simulink model "System3"  (R2025a)
settings: Solver=ode113  StartTime=0.0  StopTime=400  FixedStep=0.01  MaxStep=0.1  RelTol=1e-3
libraries: simulink x3784, slpidlib x2
(part 4 of 160)

== system System3/Battery1/Module3/SubModule_6 ==
  Module_Current : Inport
  Add : Sum  Inputs=++++++++++++++++++++++
  Add1 : Sum  Inputs=++++++++++++++++++++++
  Cell1 : Subsystem
  Cell10 : Subsystem
  Cell11 : Subsystem
  Cell12 : Subsystem
  Cell13 : Subsystem
  Cell14 : Subsystem
  Cell15 : Subsystem
  Cell16 : Subsystem
  Cell17 : Subsystem
  Cell18 : Subsystem
  Cell19 : Subsystem
  Cell2 : Subsystem
  Cell20 : Subsystem
  Cell21 : Subsystem
  Cell22 : Subsystem
  Cell3 : Subsystem
  Cell4 : Subsystem
  Cell5 : Subsystem
  Cell6 : Subsystem
  Cell7 : Subsystem
  Cell8 : Subsystem
  Cell9 : Subsystem
  Constant : Constant  Value=22
  Divide : Product  Inputs=*/
  SubModule_Voltage : Outport
  SubModule_avg_temp : Outport  Port=2
  wires:
  Cell9/2(Cell_temp) -> Add1/9
  [Cell_Current] -> Cell8/1(Cell_Current)
  Cell13/1(Cell_Voltage) -> Add/13
  Cell4/1(Cell_Voltage) -> Add/4
  Module_Current/1 -> [Cell_Current]
  Cell15/1(Cell_Voltage) -> Add/15
  [Cell_Current] -> Cell7/1(Cell_Current)
  [Cell_Current] -> Cell10/1(Cell_Current)
  Cell21/2(Cell_temp) -> Add1/21
  Cell5/1(Cell_Voltage) -> Add/5
  [Cell_Current] -> Cell1/1(Cell_Current)
  Cell2/1(Cell_Voltage) -> Add/2
  Cell19/1(Cell_Voltage) -> Add/19
  [Cell_Current] -> Cell5/1(Cell_Current)
  [Cell_Current] -> Cell11/1(Cell_Current)
  Cell6/1(Cell_Voltage) -> Add/6
  Cell11/1(Cell_Voltage) -> Add/11
  [Cell_Current] -> Cell18/1(Cell_Current)
  Cell7/2(Cell_temp) -> Add1/7
  [Cell_Current] -> Cell21/1(Cell_Current)
  [Cell_Current] -> Cell12/1(Cell_Current)
  [Cell_Current] -> Cell4/1(Cell_Current)
  Cell18/1(Cell_Voltage) -> Add/18
  Cell20/1(Cell_Voltage) -> Add/20
  Cell11/2(Cell_temp) -> Add1/11
  [Cell_Current] -> Cell2/1(Cell_Current)
  Cell16/2(Cell_temp) -> Add1/16
  [Cell_Current] -> Cell15/1(Cell_Current)
  [Cell_Current] -> Cell6/1(Cell_Current)
  [Cell_Current] -> Cell13/1(Cell_Current)
  Cell2/2(Cell_temp) -> Add1/2
  Cell22/2(Cell_temp) -> Add1/22
  Cell9/1(Cell_Voltage) -> Add/9
  Cell7/1(Cell_Voltage) -> Add/7
  [Cell_Current] -> Cell9/1(Cell_Current)
  Cell14/2(Cell_temp) -> Add1/14
  Cell17/1(Cell_Voltage) -> Add/17
  Cell10/2(Cell_temp) -> Add1/10
  [Cell_Current] -> Cell16/1(Cell_Current)
  Cell8/1(Cell_Voltage) -> Add/8
  Cell21/1(Cell_Voltage) -> Add/21
  Cell12/2(Cell_temp) -> Add1/12
  Cell22/1(Cell_Voltage) -> Add/22
  [Cell_Current] -> Cell20/1(Cell_Current)
  [Cell_Current] -> Cell17/1(Cell_Current)
  Cell10/1(Cell_Voltage) -> Add/10
  Cell18/2(Cell_temp) -> Add1/18
  Cell14/1(Cell_Voltage) -> Add/14
  Cell16/1(Cell_Voltage) -> Add/16
  [Cell_Current] -> Cell3/1(Cell_Current)
  Cell12/1(Cell_Voltage) -> Add/12
  Cell20/2(Cell_temp) -> Add1/20
  Cell1/1(Cell_Voltage) -> Add/1
  [Cell_Current] -> Cell19/1(Cell_Current)
  Cell3/1(Cell_Voltage) -> Add/3
  [Cell_Current] -> Cell22/1(Cell_Current)
  [Cell_Current] -> Cell14/1(Cell_Current)
  Cell19/2(Cell_temp) -> Add1/19
  Cell6/2(Cell_temp) -> Add1/6
  Cell17/2(Cell_temp) -> Add1/17
  Cell15/2(Cell_temp) -> Add1/15
  Cell8/2(Cell_temp) -> Add1/8
  Cell3/2(Cell_temp) -> Add1/3
  Cell13/2(Cell_temp) -> Add1/13
  Add/1 -> SubModule_Voltage/1
  Cell4/2(Cell_temp) -> Add1/4
  Cell5/2(Cell_temp) -> Add1/5
  Cell1/2(Cell_temp) -> Add1/1
  Add1/1 -> Divide/1
  Constant/1 -> Divide/2
  Divide/1 -> SubModule_avg_temp/1

== system System3/Battery1/Module3/SubModule_7 ==
  Module_Current : Inport
  Add : Sum  Inputs=++++++++++++++++++++++
  Add1 : Sum  Inputs=++++++++++++++++++++++
  Cell1 : Subsystem
  Cell10 : Subsystem
  Cell11 : Subsystem
  Cell12 : Subsystem
  Cell13 : Subsystem
  Cell14 : Subsystem
  Cell15 : Subsystem
  Cell16 : Subsystem
  Cell17 : Subsystem
  Cell18 : Subsystem
  Cell19 : Subsystem
  Cell2 : Subsystem
  Cell20 : Subsystem
  Cell21 : Subsystem
  Cell22 : Subsystem
  Cell3 : Subsystem
  Cell4 : Subsystem
  Cell5 : Subsystem
  Cell6 : Subsystem
  Cell7 : Subsystem
  Cell8 : Subsystem
  Cell9 : Subsystem
  Constant : Constant  Value=22
  Divide : Product  Inputs=*/
  SubModule_Voltage : Outport
  SubModule_avg_temp : Outport  Port=2
  wires:
  Cell9/2(Cell_temp) -> Add1/9
  [Cell_Current] -> Cell8/1(Cell_Current)
  Cell13/1(Cell_Voltage) -> Add/13
  Cell4/1(Cell_Voltage) -> Add/4
  Module_Current/1 -> [Cell_Current]
  Cell15/1(Cell_Voltage) -> Add/15
  [Cell_Current] -> Cell7/1(Cell_Current)
  [Cell_Current] -> Cell10/1(Cell_Current)
  Cell21/2(Cell_temp) -> Add1/21
  Cell5/1(Cell_Voltage) -> Add/5
  [Cell_Current] -> Cell1/1(Cell_Current)
  Cell2/1(Cell_Voltage) -> Add/2
  Cell19/1(Cell_Voltage) -> Add/19
  [Cell_Current] -> Cell5/1(Cell_Current)
  [Cell_Current] -> Cell11/1(Cell_Current)
  Cell6/1(Cell_Voltage) -> Add/6
  Cell11/1(Cell_Voltage) -> Add/11
  [Cell_Current] -> Cell18/1(Cell_Current)
  Cell7/2(Cell_temp) -> Add1/7
  [Cell_Current] -> Cell21/1(Cell_Current)
  [Cell_Current] -> Cell12/1(Cell_Current)
  [Cell_Current] -> Cell4/1(Cell_Current)
  Cell18/1(Cell_Voltage) -> Add/18
  Cell20/1(Cell_Voltage) -> Add/20
  Cell11/2(Cell_temp) -> Add1/11
  [Cell_Current] -> Cell2/1(Cell_Current)
  Cell16/2(Cell_temp) -> Add1/16
  [Cell_Current] -> Cell15/1(Cell_Current)
  [Cell_Current] -> Cell6/1(Cell_Current)
  [Cell_Current] -> Cell13/1(Cell_Current)
  Cell2/2(Cell_temp) -> Add1/2
  Cell22/2(Cell_temp) -> Add1/22
  Cell9/1(Cell_Voltage) -> Add/9
  Cell7/1(Cell_Voltage) -> Add/7
  [Cell_Current] -> Cell9/1(Cell_Current)
  Cell14/2(Cell_temp) -> Add1/14
  Cell17/1(Cell_Voltage) -> Add/17
  Cell10/2(Cell_temp) -> Add1/10
  [Cell_Current] -> Cell16/1(Cell_Current)
  Cell8/1(Cell_Voltage) -> Add/8
  Cell21/1(Cell_Voltage) -> Add/21
  Cell12/2(Cell_temp) -> Add1/12
  Cell22/1(Cell_Voltage) -> Add/22
  [Cell_Current] -> Cell20/1(Cell_Current)
  [Cell_Current] -> Cell17/1(Cell_Current)
  Cell10/1(Cell_Voltage) -> Add/10
  Cell18/2(Cell_temp) -> Add1/18
  Cell14/1(Cell_Voltage) -> Add/14
  Cell16/1(Cell_Voltage) -> Add/16
  [Cell_Current] -> Cell3/1(Cell_Current)
  Cell12/1(Cell_Voltage) -> Add/12
  Cell20/2(Cell_temp) -> Add1/20
  Cell1/1(Cell_Voltage) -> Add/1
  [Cell_Current] -> Cell19/1(Cell_Current)
  Cell3/1(Cell_Voltage) -> Add/3
  [Cell_Current] -> Cell22/1(Cell_Current)
  [Cell_Current] -> Cell14/1(Cell_Current)
  Cell19/2(Cell_temp) -> Add1/19
  Cell6/2(Cell_temp) -> Add1/6
  Cell17/2(Cell_temp) -> Add1/17
  Cell15/2(Cell_temp) -> Add1/15
  Cell8/2(Cell_temp) -> Add1/8
  Cell3/2(Cell_temp) -> Add1/3
  Cell13/2(Cell_temp) -> Add1/13
  Add/1 -> SubModule_Voltage/1
  Cell4/2(Cell_temp) -> Add1/4
  Cell5/2(Cell_temp) -> Add1/5
  Cell1/2(Cell_temp) -> Add1/1
  Add1/1 -> Divide/1
  Constant/1 -> Divide/2
  Divide/1 -> SubModule_avg_temp/1

== system System3/Battery1/Module3/SubModule_8 ==
  Module_Current : Inport
  Add : Sum  Inputs=++++++++++++++++++++++
  Add1 : Sum  Inputs=++++++++++++++++++++++
  Cell1 : Subsystem
  Cell10 : Subsystem
  Cell11 : Subsystem
  Cell12 : Subsystem
  Cell13 : Subsystem
  Cell14 : Subsystem
  Cell15 : Subsystem
  Cell16 : Subsystem
  Cell17 : Subsystem
  Cell18 : Subsystem
  Cell19 : Subsystem
  Cell2 : Subsystem
  Cell20 : Subsystem
  Cell21 : Subsystem
  Cell22 : Subsystem
  Cell3 : Subsystem
  Cell4 : Subsystem
  Cell5 : Subsystem
  Cell6 : Subsystem
  Cell7 : Subsystem
  Cell8 : Subsystem
  Cell9 : Subsystem
  Constant : Constant  Value=22
  Divide : Product  Inputs=*/
  SubModule_Voltage : Outport
  SubModule_avg_temp : Outport  Port=2
  wires:
  Divide/1 -> SubModule_avg_temp/1
  Constant/1 -> Divide/2
  Add1/1 -> Divide/1
  Cell1/2(Cell_temp) -> Add1/1
  Cell5/2(Cell_temp) -> Add1/5
  Cell4/2(Cell_temp) -> Add1/4
  Add/1 -> SubModule_Voltage/1
  Cell13/2(Cell_temp) -> Add1/13
  Cell3/2(Cell_temp) -> Add1/3
  Cell8/2(Cell_temp) -> Add1/8
  Cell15/2(Cell_temp) -> Add1/15
  Cell17/2(Cell_temp) -> Add1/17
  Cell6/2(Cell_temp) -> Add1/6
  Cell19/2(Cell_temp) -> Add1/19
  [Cell_Current] -> Cell14/1(Cell_Current)
  [Cell_Current] -> Cell22/1(Cell_Current)
  Cell3/1(Cell_Voltage) -> Add/3
  [Cell_Current] -> Cell19/1(Cell_Current)
  Cell1/1(Cell_Voltage) -> Add/1
  Cell20/2(Cell_temp) -> Add1/20
  Cell12/1(Cell_Voltage) -> Add/12
  [Cell_Current] -> Cell3/1(Cell_Current)
  Cell16/1(Cell_Voltage) -> Add/16
  Cell14/1(Cell_Voltage) -> Add/14
  Cell18/2(Cell_temp) -> Add1/18
  Cell10/1(Cell_Voltage) -> Add/10
  [Cell_Current] -> Cell17/1(Cell_Current)
  [Cell_Current] -> Cell20/1(Cell_Current)
  Cell22/1(Cell_Voltage) -> Add/22
  Cell12/2(Cell_temp) -> Add1/12
  Cell21/1(Cell_Voltage) -> Add/21
  Cell8/1(Cell_Voltage) -> Add/8
  [Cell_Current] -> Cell16/1(Cell_Current)
  Cell10/2(Cell_temp) -> Add1/10
  Cell17/1(Cell_Voltage) -> Add/17
  Cell14/2(Cell_temp) -> Add1/14
  [Cell_Current] -> Cell9/1(Cell_Current)
  Cell7/1(Cell_Voltage) -> Add/7
  Cell9/1(Cell_Voltage) -> Add/9
  Cell22/2(Cell_temp) -> Add1/22
  Cell2/2(Cell_temp) -> Add1/2
  [Cell_Current] -> Cell13/1(Cell_Current)
  [Cell_Current] -> Cell6/1(Cell_Current)
  [Cell_Current] -> Cell15/1(Cell_Current)
  Cell16/2(Cell_temp) -> Add1/16
  [Cell_Current] -> Cell2/1(Cell_Current)
  Cell11/2(Cell_temp) -> Add1/11
  Cell20/1(Cell_Voltage) -> Add/20
  Cell18/1(Cell_Voltage) -> Add/18
  [Cell_Current] -> Cell4/1(Cell_Current)
  [Cell_Current] -> Cell12/1(Cell_Current)
  [Cell_Current] -> Cell21/1(Cell_Current)
  Cell7/2(Cell_temp) -> Add1/7
  [Cell_Current] -> Cell18/1(Cell_Current)
  Cell11/1(Cell_Voltage) -> Add/11
  Cell6/1(Cell_Voltage) -> Add/6
  [Cell_Current] -> Cell11/1(Cell_Current)
  [Cell_Current] -> Cell5/1(Cell_Current)
  Cell19/1(Cell_Voltage) -> Add/19
  Cell2/1(Cell_Voltage) -> Add/2
  [Cell_Current] -> Cell1/1(Cell_Current)
  Cell5/1(Cell_Voltage) -> Add/5
  Cell21/2(Cell_temp) -> Add1/21
  [Cell_Current] -> Cell10/1(Cell_Current)
  [Cell_Current] -> Cell7/1(Cell_Current)
  Cell15/1(Cell_Voltage) -> Add/15
  Module_Current/1 -> [Cell_Current]
  Cell4/1(Cell_Voltage) -> Add/4
  Cell13/1(Cell_Voltage) -> Add/13
  [Cell_Current] -> Cell8/1(Cell_Current)
  Cell9/2(Cell_temp) -> Add1/9

== system System3/Battery1/Module3/SubModule_9 ==
  Module_Current : Inport
  Add : Sum  Inputs=++++++++++++++++++++++
  Add1 : Sum  Inputs=++++++++++++++++++++++
  Cell1 : Subsystem
  Cell10 : Subsystem
  Cell11 : Subsystem
  Cell12 : Subsystem
  Cell13 : Subsystem
  Cell14 : Subsystem
  Cell15 : Subsystem
  Cell16 : Subsystem
  Cell17 : Subsystem
  Cell18 : Subsystem
  Cell19 : Subsystem
  Cell2 : Subsystem
  Cell20 : Subsystem
  Cell21 : Subsystem
  Cell22 : Subsystem
  Cell3 : Subsystem
  Cell4 : Subsystem
  Cell5 : Subsystem
  Cell6 : Subsystem
  Cell7 : Subsystem
  Cell8 : Subsystem
  Cell9 : Subsystem
  Constant : Constant  Value=22
  Divide : Product  Inputs=*/
  SubModule_Voltage : Outport
  SubModule_avg_temp : Outport  Port=2
  wires:
  Cell9/2(Cell_temp) -> Add1/9
  [Cell_Current] -> Cell8/1(Cell_Current)
  Cell13/1(Cell_Voltage) -> Add/13
  Cell4/1(Cell_Voltage) -> Add/4
  Module_Current/1 -> [Cell_Current]
  Cell15/1(Cell_Voltage) -> Add/15
  [Cell_Current] -> Cell7/1(Cell_Current)
  [Cell_Current] -> Cell10/1(Cell_Current)
  Cell21/2(Cell_temp) -> Add1/21
  Cell5/1(Cell_Voltage) -> Add/5
  [Cell_Current] -> Cell1/1(Cell_Current)
  Cell2/1(Cell_Voltage) -> Add/2
  Cell19/1(Cell_Voltage) -> Add/19
  [Cell_Current] -> Cell5/1(Cell_Current)
  [Cell_Current] -> Cell11/1(Cell_Current)
  Cell6/1(Cell_Voltage) -> Add/6
  Cell11/1(Cell_Voltage) -> Add/11
  [Cell_Current] -> Cell18/1(Cell_Current)
  Cell7/2(Cell_temp) -> Add1/7
  [Cell_Current] -> Cell21/1(Cell_Current)
  [Cell_Current] -> Cell12/1(Cell_Current)
  [Cell_Current] -> Cell4/1(Cell_Current)
  Cell18/1(Cell_Voltage) -> Add/18
  Cell20/1(Cell_Voltage) -> Add/20
  Cell11/2(Cell_temp) -> Add1/11
  [Cell_Current] -> Cell2/1(Cell_Current)
  Cell16/2(Cell_temp) -> Add1/16
  [Cell_Current] -> Cell15/1(Cell_Current)
  [Cell_Current] -> Cell6/1(Cell_Current)
  [Cell_Current] -> Cell13/1(Cell_Current)
  Cell2/2(Cell_temp) -> Add1/2
  Cell22/2(Cell_temp) -> Add1/22
  Cell9/1(Cell_Voltage) -> Add/9
  Cell7/1(Cell_Voltage) -> Add/7
  [Cell_Current] -> Cell9/1(Cell_Current)
  Cell14/2(Cell_temp) -> Add1/14
  Cell17/1(Cell_Voltage) -> Add/17
  Cell10/2(Cell_temp) -> Add1/10
  [Cell_Current] -> Cell16/1(Cell_Current)
  Cell8/1(Cell_Voltage) -> Add/8
  Cell21/1(Cell_Voltage) -> Add/21
  Cell12/2(Cell_temp) -> Add1/12
  Cell22/1(Cell_Voltage) -> Add/22
  [Cell_Current] -> Cell20/1(Cell_Current)
  [Cell_Current] -> Cell17/1(Cell_Current)
  Cell10/1(Cell_Voltage) -> Add/10
  Cell18/2(Cell_temp) -> Add1/18
  Cell14/1(Cell_Voltage) -> Add/14
  Cell16/1(Cell_Voltage) -> Add/16
  [Cell_Current] -> Cell3/1(Cell_Current)
  Cell12/1(Cell_Voltage) -> Add/12
  Cell20/2(Cell_temp) -> Add1/20
  Cell1/1(Cell_Voltage) -> Add/1
  [Cell_Current] -> Cell19/1(Cell_Current)
  Cell3/1(Cell_Voltage) -> Add/3
  [Cell_Current] -> Cell22/1(Cell_Current)
  [Cell_Current] -> Cell14/1(Cell_Current)
  Cell19/2(Cell_temp) -> Add1/19
  Cell6/2(Cell_temp) -> Add1/6
  Cell17/2(Cell_temp) -> Add1/17
  Cell15/2(Cell_temp) -> Add1/15
  Cell8/2(Cell_temp) -> Add1/8
  Cell3/2(Cell_temp) -> Add1/3
  Cell13/2(Cell_temp) -> Add1/13
  Add/1 -> SubModule_Voltage/1
  Cell4/2(Cell_temp) -> Add1/4
  Cell5/2(Cell_temp) -> Add1/5
  Cell1/2(Cell_temp) -> Add1/1
  Add1/1 -> Divide/1
  Constant/1 -> Divide/2
  Divide/1 -> SubModule_avg_temp/1

== system System3/Battery1/SOCEstimator/SOCEstimator ==
  SOC_Initial : Inport
  Current : Inport  Port=2
  CellCapacity : Inport  Port=3
  Add1 : Sum  Inputs=+-
  Constant : Constant  Value=100  SampleTime=-1
  Constant1 : Constant  Value=3600  SampleTime=-1
  Delay : Delay  DelayLength=1  InitialConditionSource=Input port
      settings: InputPortMap=u0,p4
  Divide : Product  Inputs=*//
  Divide1 : Product  Inputs=*/
  Integrator : Integrator
  Saturation1 : Saturate  UpperLimit=1  LowerLimit=0
  SOC : Outport
  wires:
  Add1/1 -> Saturation1/1
  Constant/1 -> Divide1/2
  Divide1/1 -> Delay/2, Add1/1
  Divide/1 -> Add1/2
  Saturation1/1 -> Delay/1
  SOC_Initial/1 -> Divide1/1
  Current/1 -> Integrator/1
  Delay/1 -> SOC/1
  CellCapacity/1 -> Divide/2
  Constant1/1 -> Divide/3
  Integrator/1 -> Divide/1

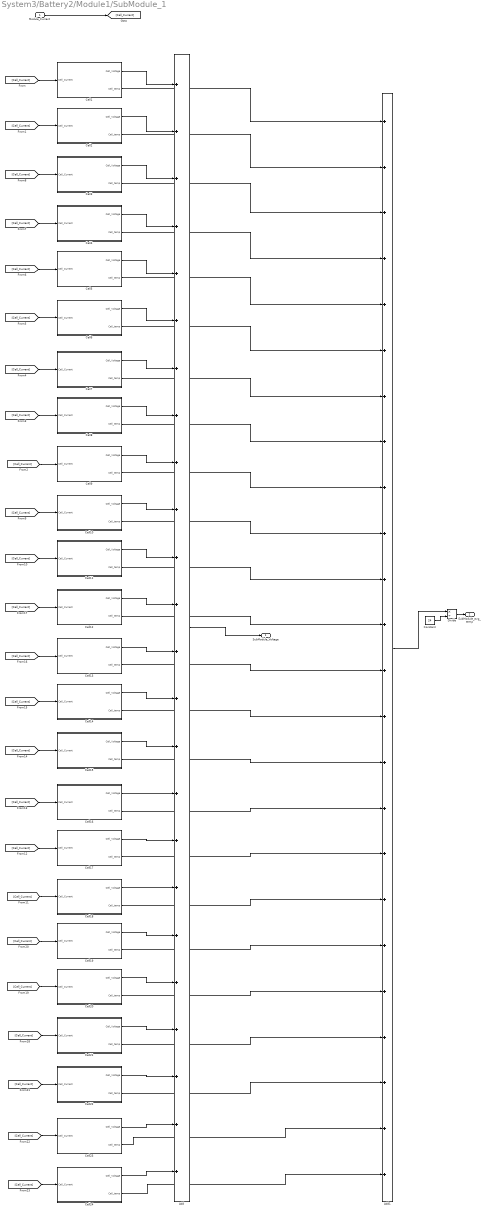
== system System3/Battery2/Module1/SubModule_1 ==
  Module_Current : Inport
  Add : Sum  Inputs=++++++++++++++++++++++++
  Add1 : Sum  Inputs=++++++++++++++++++++++++
  Cell1 : Subsystem
  Cell10 : Subsystem
  Cell11 : Subsystem
  Cell12 : Subsystem
  Cell13 : Subsystem
  Cell14 : Subsystem
  Cell15 : Subsystem
  Cell16 : Subsystem
  Cell17 : Subsystem
  Cell18 : Subsystem
  Cell19 : Subsystem
  Cell2 : Subsystem
  Cell20 : Subsystem
  Cell21 : Subsystem
  Cell22 : Subsystem
  Cell23 : Subsystem
  Cell24 : Subsystem
  Cell3 : Subsystem
  Cell4 : Subsystem
  Cell5 : Subsystem
  Cell6 : Subsystem
  Cell7 : Subsystem
  Cell8 : Subsystem
  Cell9 : Subsystem
  Constant : Constant  Value=24
  Divide : Product  Inputs=*/
  SubModule_Voltage : Outport
  SubModule_avg_temp : Outport  Port=2
  wires:
  Cell9/2(Cell_temp) -> Add1/9
  [Cell_Current] -> Cell8/1(Cell_Current)
  Cell13/1(Cell_Voltage) -> Add/13
  Cell4/1(Cell_Voltage) -> Add/4
  Module_Current/1 -> [Cell_Current]
  Cell15/1(Cell_Voltage) -> Add/15
  [Cell_Current] -> Cell7/1(Cell_Current)
  [Cell_Current] -> Cell10/1(Cell_Current)
  Cell21/2(Cell_temp) -> Add1/21
  Cell5/1(Cell_Voltage) -> Add/5
  [Cell_Current] -> Cell1/1(Cell_Current)
  Cell2/1(Cell_Voltage) -> Add/2
  Cell19/1(Cell_Voltage) -> Add/19
  [Cell_Current] -> Cell5/1(Cell_Current)
  [Cell_Current] -> Cell11/1(Cell_Current)
  Cell6/1(Cell_Voltage) -> Add/6
  Cell11/1(Cell_Voltage) -> Add/11
  [Cell_Current] -> Cell18/1(Cell_Current)
  Cell7/2(Cell_temp) -> Add1/7
  [Cell_Current] -> Cell21/1(Cell_Current)
  [Cell_Current] -> Cell12/1(Cell_Current)
  [Cell_Current] -> Cell4/1(Cell_Current)
  Cell18/1(Cell_Voltage) -> Add/18
  Cell20/1(Cell_Voltage) -> Add/20
  Cell11/2(Cell_temp) -> Add1/11
  [Cell_Current] -> Cell2/1(Cell_Current)
  Cell16/2(Cell_temp) -> Add1/16
  [Cell_Current] -> Cell15/1(Cell_Current)
  [Cell_Current] -> Cell6/1(Cell_Current)
  [Cell_Current] -> Cell13/1(Cell_Current)
  Cell2/2(Cell_temp) -> Add1/2
  Cell22/2(Cell_temp) -> Add1/22
  Cell9/1(Cell_Voltage) -> Add/9
  Cell7/1(Cell_Voltage) -> Add/7
  [Cell_Current] -> Cell9/1(Cell_Current)
  Cell14/2(Cell_temp) -> Add1/14
  Cell17/1(Cell_Voltage) -> Add/17
  Cell10/2(Cell_temp) -> Add1/10
  [Cell_Current] -> Cell16/1(Cell_Current)
  Cell8/1(Cell_Voltage) -> Add/8
  Cell21/1(Cell_Voltage) -> Add/21
  Cell12/2(Cell_temp) -> Add1/12
  Cell22/1(Cell_Voltage) -> Add/22
  [Cell_Current] -> Cell20/1(Cell_Current)
  [Cell_Current] -> Cell17/1(Cell_Current)
  Cell10/1(Cell_Voltage) -> Add/10
  Cell18/2(Cell_temp) -> Add1/18
  Cell14/1(Cell_Voltage) -> Add/14
  Cell16/1(Cell_Voltage) -> Add/16
  [Cell_Current] -> Cell3/1(Cell_Current)
  Cell12/1(Cell_Voltage) -> Add/12
  Cell20/2(Cell_temp) -> Add1/20
  Cell1/1(Cell_Voltage) -> Add/1
  [Cell_Current] -> Cell19/1(Cell_Current)
  Cell3/1(Cell_Voltage) -> Add/3
  [Cell_Current] -> Cell22/1(Cell_Current)
  [Cell_Current] -> Cell14/1(Cell_Current)
  Cell19/2(Cell_temp) -> Add1/19
  Cell6/2(Cell_temp) -> Add1/6
  Cell17/2(Cell_temp) -> Add1/17
  Cell15/2(Cell_temp) -> Add1/15
  Cell8/2(Cell_temp) -> Add1/8
  Cell3/2(Cell_temp) -> Add1/3
  Cell13/2(Cell_temp) -> Add1/13
  Add/1 -> SubModule_Voltage/1
  Cell4/2(Cell_temp) -> Add1/4
  Cell5/2(Cell_temp) -> Add1/5
  Cell1/2(Cell_temp) -> Add1/1
  Add1/1 -> Divide/1
  Constant/1 -> Divide/2
  Divide/1 -> SubModule_avg_temp/1
  [Cell_Current] -> Cell24/1(Cell_Current)
  [Cell_Current] -> Cell23/1(Cell_Current)
  Cell23/1(Cell_Voltage) -> Add/23
  Cell24/1(Cell_Voltage) -> Add/24
  Cell23/2(Cell_temp) -> Add1/23
  Cell24/2(Cell_temp) -> Add1/24

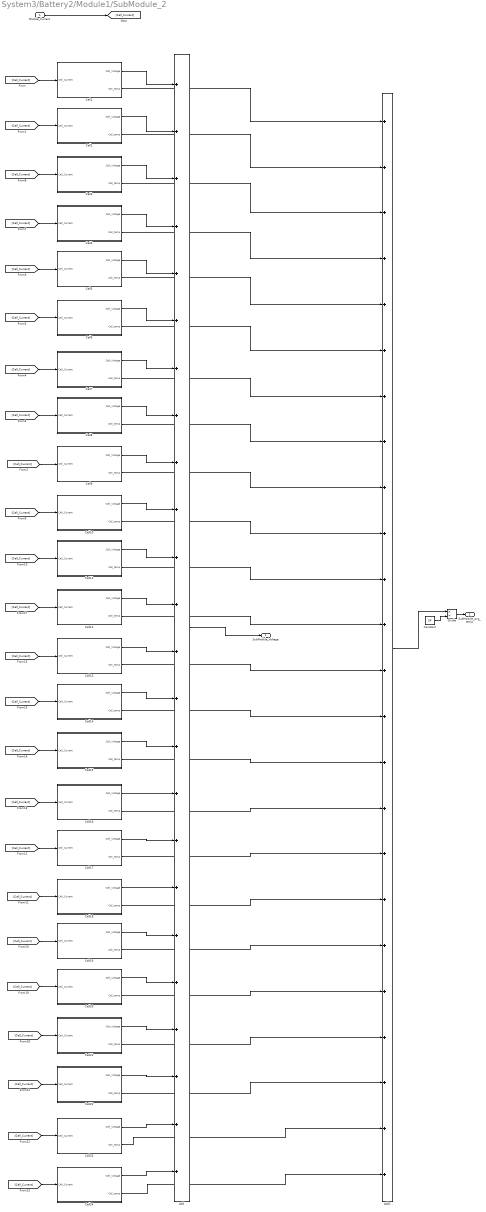
== system System3/Battery2/Module1/SubModule_2 ==
  Module_Current : Inport
  Add : Sum  Inputs=++++++++++++++++++++++++
  Add1 : Sum  Inputs=++++++++++++++++++++++++
  Cell1 : Subsystem
  Cell10 : Subsystem
  Cell11 : Subsystem
  Cell12 : Subsystem
  Cell13 : Subsystem
  Cell14 : Subsystem
  Cell15 : Subsystem
  Cell16 : Subsystem
  Cell17 : Subsystem
  Cell18 : Subsystem
  Cell19 : Subsystem
  Cell2 : Subsystem
  Cell20 : Subsystem
  Cell21 : Subsystem
  Cell22 : Subsystem
  Cell23 : Subsystem
  Cell24 : Subsystem
  Cell3 : Subsystem
  Cell4 : Subsystem
  Cell5 : Subsystem
  Cell6 : Subsystem
  Cell7 : Subsystem
  Cell8 : Subsystem
  Cell9 : Subsystem
  Constant : Constant  Value=24
  Divide : Product  Inputs=*/
  SubModule_Voltage : Outport
  SubModule_avg_temp : Outport  Port=2
  wires:
  Cell24/2(Cell_temp) -> Add1/24
  Cell23/2(Cell_temp) -> Add1/23
  Cell24/1(Cell_Voltage) -> Add/24
  Cell23/1(Cell_Voltage) -> Add/23
  [Cell_Current] -> Cell23/1(Cell_Current)
  [Cell_Current] -> Cell24/1(Cell_Current)
  Divide/1 -> SubModule_avg_temp/1
  Constant/1 -> Divide/2
  Add1/1 -> Divide/1
  Cell1/2(Cell_temp) -> Add1/1
  Cell5/2(Cell_temp) -> Add1/5
  Cell4/2(Cell_temp) -> Add1/4
  Add/1 -> SubModule_Voltage/1
  Cell13/2(Cell_temp) -> Add1/13
  Cell3/2(Cell_temp) -> Add1/3
  Cell8/2(Cell_temp) -> Add1/8
  Cell15/2(Cell_temp) -> Add1/15
  Cell17/2(Cell_temp) -> Add1/17
  Cell6/2(Cell_temp) -> Add1/6
  Cell19/2(Cell_temp) -> Add1/19
  [Cell_Current] -> Cell14/1(Cell_Current)
  [Cell_Current] -> Cell22/1(Cell_Current)
  Cell3/1(Cell_Voltage) -> Add/3
  [Cell_Current] -> Cell19/1(Cell_Current)
  Cell1/1(Cell_Voltage) -> Add/1
  Cell20/2(Cell_temp) -> Add1/20
  Cell12/1(Cell_Voltage) -> Add/12
  [Cell_Current] -> Cell3/1(Cell_Current)
  Cell16/1(Cell_Voltage) -> Add/16
  Cell14/1(Cell_Voltage) -> Add/14
  Cell18/2(Cell_temp) -> Add1/18
  Cell10/1(Cell_Voltage) -> Add/10
  [Cell_Current] -> Cell17/1(Cell_Current)
  [Cell_Current] -> Cell20/1(Cell_Current)
  Cell22/1(Cell_Voltage) -> Add/22
  Cell12/2(Cell_temp) -> Add1/12
  Cell21/1(Cell_Voltage) -> Add/21
  Cell8/1(Cell_Voltage) -> Add/8
  [Cell_Current] -> Cell16/1(Cell_Current)
  Cell10/2(Cell_temp) -> Add1/10
  Cell17/1(Cell_Voltage) -> Add/17
  Cell14/2(Cell_temp) -> Add1/14
  [Cell_Current] -> Cell9/1(Cell_Current)
  Cell7/1(Cell_Voltage) -> Add/7
  Cell9/1(Cell_Voltage) -> Add/9
  Cell22/2(Cell_temp) -> Add1/22
  Cell2/2(Cell_temp) -> Add1/2
  [Cell_Current] -> Cell13/1(Cell_Current)
  [Cell_Current] -> Cell6/1(Cell_Current)
  [Cell_Current] -> Cell15/1(Cell_Current)
  Cell16/2(Cell_temp) -> Add1/16
  [Cell_Current] -> Cell2/1(Cell_Current)
  Cell11/2(Cell_temp) -> Add1/11
  Cell20/1(Cell_Voltage) -> Add/20
  Cell18/1(Cell_Voltage) -> Add/18
  [Cell_Current] -> Cell4/1(Cell_Current)
  [Cell_Current] -> Cell12/1(Cell_Current)
  [Cell_Current] -> Cell21/1(Cell_Current)
  Cell7/2(Cell_temp) -> Add1/7
  [Cell_Current] -> Cell18/1(Cell_Current)
  Cell11/1(Cell_Voltage) -> Add/11
  Cell6/1(Cell_Voltage) -> Add/6
  [Cell_Current] -> Cell11/1(Cell_Current)
  [Cell_Current] -> Cell5/1(Cell_Current)
  Cell19/1(Cell_Voltage) -> Add/19
  Cell2/1(Cell_Voltage) -> Add/2
  [Cell_Current] -> Cell1/1(Cell_Current)
  Cell5/1(Cell_Voltage) -> Add/5
  Cell21/2(Cell_temp) -> Add1/21
  [Cell_Current] -> Cell10/1(Cell_Current)
  [Cell_Current] -> Cell7/1(Cell_Current)
  Cell15/1(Cell_Voltage) -> Add/15
  Module_Current/1 -> [Cell_Current]
  Cell4/1(Cell_Voltage) -> Add/4
  Cell13/1(Cell_Voltage) -> Add/13
  [Cell_Current] -> Cell8/1(Cell_Current)
  Cell9/2(Cell_temp) -> Add1/9

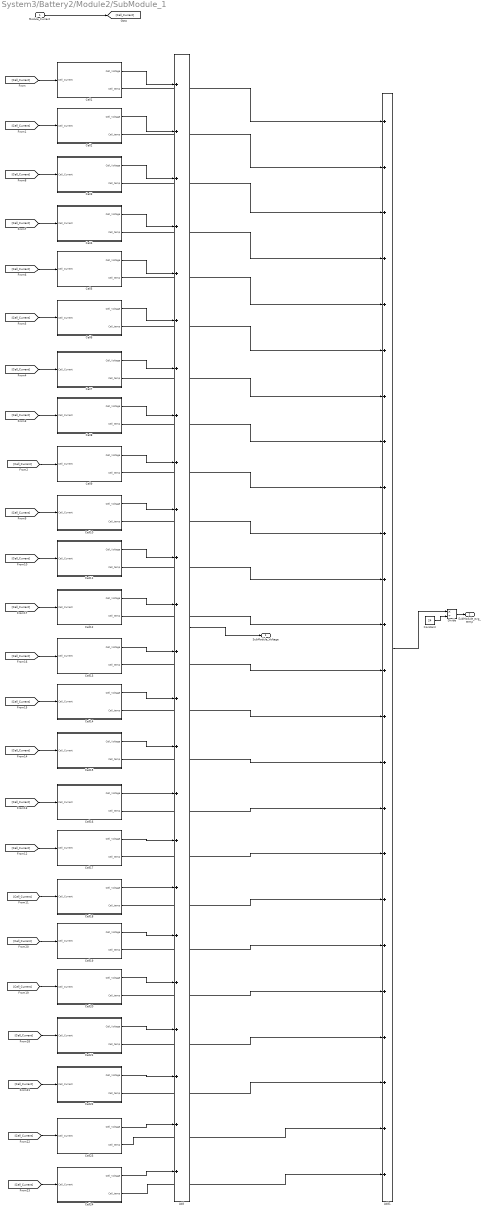
== system System3/Battery2/Module2/SubModule_1 ==
  Module_Current : Inport
  Add : Sum  Inputs=++++++++++++++++++++++++
  Add1 : Sum  Inputs=++++++++++++++++++++++++
  Cell1 : Subsystem
  Cell10 : Subsystem
  Cell11 : Subsystem
  Cell12 : Subsystem
  Cell13 : Subsystem
  Cell14 : Subsystem
  Cell15 : Subsystem
  Cell16 : Subsystem
  Cell17 : Subsystem
  Cell18 : Subsystem
  Cell19 : Subsystem
  Cell2 : Subsystem
  Cell20 : Subsystem
  Cell21 : Subsystem
  Cell22 : Subsystem
  Cell23 : Subsystem
  Cell24 : Subsystem
  Cell3 : Subsystem
  Cell4 : Subsystem
  Cell5 : Subsystem
  Cell6 : Subsystem
  Cell7 : Subsystem
  Cell8 : Subsystem
  Cell9 : Subsystem
  Constant : Constant  Value=24
  Divide : Product  Inputs=*/
  SubModule_Voltage : Outport
  SubModule_avg_temp : Outport  Port=2
  wires:
  Cell24/2(Cell_temp) -> Add1/24
  Cell23/2(Cell_temp) -> Add1/23
  Cell24/1(Cell_Voltage) -> Add/24
  Cell23/1(Cell_Voltage) -> Add/23
  [Cell_Current] -> Cell23/1(Cell_Current)
  [Cell_Current] -> Cell24/1(Cell_Current)
  Divide/1 -> SubModule_avg_temp/1
  Constant/1 -> Divide/2
  Add1/1 -> Divide/1
  Cell1/2(Cell_temp) -> Add1/1
  Cell5/2(Cell_temp) -> Add1/5
  Cell4/2(Cell_temp) -> Add1/4
  Add/1 -> SubModule_Voltage/1
  Cell13/2(Cell_temp) -> Add1/13
  Cell3/2(Cell_temp) -> Add1/3
  Cell8/2(Cell_temp) -> Add1/8
  Cell15/2(Cell_temp) -> Add1/15
  Cell17/2(Cell_temp) -> Add1/17
  Cell6/2(Cell_temp) -> Add1/6
  Cell19/2(Cell_temp) -> Add1/19
  [Cell_Current] -> Cell14/1(Cell_Current)
  [Cell_Current] -> Cell22/1(Cell_Current)
  Cell3/1(Cell_Voltage) -> Add/3
  [Cell_Current] -> Cell19/1(Cell_Current)
  Cell1/1(Cell_Voltage) -> Add/1
  Cell20/2(Cell_temp) -> Add1/20
  Cell12/1(Cell_Voltage) -> Add/12
  [Cell_Current] -> Cell3/1(Cell_Current)
  Cell16/1(Cell_Voltage) -> Add/16
  Cell14/1(Cell_Voltage) -> Add/14
  Cell18/2(Cell_temp) -> Add1/18
  Cell10/1(Cell_Voltage) -> Add/10
  [Cell_Current] -> Cell17/1(Cell_Current)
  [Cell_Current] -> Cell20/1(Cell_Current)
  Cell22/1(Cell_Voltage) -> Add/22
  Cell12/2(Cell_temp) -> Add1/12
  Cell21/1(Cell_Voltage) -> Add/21
  Cell8/1(Cell_Voltage) -> Add/8
  [Cell_Current] -> Cell16/1(Cell_Current)
  Cell10/2(Cell_temp) -> Add1/10
  Cell17/1(Cell_Voltage) -> Add/17
  Cell14/2(Cell_temp) -> Add1/14
  [Cell_Current] -> Cell9/1(Cell_Current)
  Cell7/1(Cell_Voltage) -> Add/7
  Cell9/1(Cell_Voltage) -> Add/9
  Cell22/2(Cell_temp) -> Add1/22
  Cell2/2(Cell_temp) -> Add1/2
  [Cell_Current] -> Cell13/1(Cell_Current)
  [Cell_Current] -> Cell6/1(Cell_Current)
  [Cell_Current] -> Cell15/1(Cell_Current)
  Cell16/2(Cell_temp) -> Add1/16
  [Cell_Current] -> Cell2/1(Cell_Current)
  Cell11/2(Cell_temp) -> Add1/11
  Cell20/1(Cell_Voltage) -> Add/20
  Cell18/1(Cell_Voltage) -> Add/18
  [Cell_Current] -> Cell4/1(Cell_Current)
  [Cell_Current] -> Cell12/1(Cell_Current)
  [Cell_Current] -> Cell21/1(Cell_Current)
  Cell7/2(Cell_temp) -> Add1/7
  [Cell_Current] -> Cell18/1(Cell_Current)
  Cell11/1(Cell_Voltage) -> Add/11
  Cell6/1(Cell_Voltage) -> Add/6
  [Cell_Current] -> Cell11/1(Cell_Current)
  [Cell_Current] -> Cell5/1(Cell_Current)
  Cell19/1(Cell_Voltage) -> Add/19
  Cell2/1(Cell_Voltage) -> Add/2
  [Cell_Current] -> Cell1/1(Cell_Current)
  Cell5/1(Cell_Voltage) -> Add/5
  Cell21/2(Cell_temp) -> Add1/21
  [Cell_Current] -> Cell10/1(Cell_Current)
  [Cell_Current] -> Cell7/1(Cell_Current)
  Cell15/1(Cell_Voltage) -> Add/15
  Module_Current/1 -> [Cell_Current]
  Cell4/1(Cell_Voltage) -> Add/4
  Cell13/1(Cell_Voltage) -> Add/13
  [Cell_Current] -> Cell8/1(Cell_Current)
  Cell9/2(Cell_temp) -> Add1/9

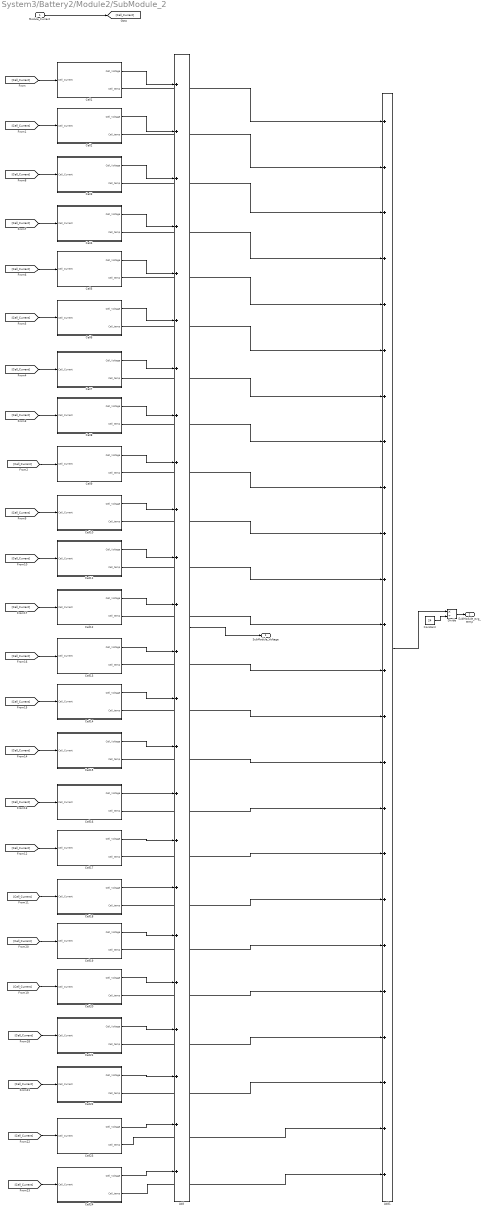
== system System3/Battery2/Module2/SubModule_2 ==
  Module_Current : Inport
  Add : Sum  Inputs=++++++++++++++++++++++++
  Add1 : Sum  Inputs=++++++++++++++++++++++++
  Cell1 : Subsystem
  Cell10 : Subsystem
  Cell11 : Subsystem
  Cell12 : Subsystem
  Cell13 : Subsystem
  Cell14 : Subsystem
  Cell15 : Subsystem
  Cell16 : Subsystem
  Cell17 : Subsystem
  Cell18 : Subsystem
  Cell19 : Subsystem
  Cell2 : Subsystem
  Cell20 : Subsystem
  Cell21 : Subsystem
  Cell22 : Subsystem
  Cell23 : Subsystem
  Cell24 : Subsystem
  Cell3 : Subsystem
  Cell4 : Subsystem
  Cell5 : Subsystem
  Cell6 : Subsystem
  Cell7 : Subsystem
  Cell8 : Subsystem
  Cell9 : Subsystem
  Constant : Constant  Value=24
  Divide : Product  Inputs=*/
  SubModule_Voltage : Outport
  SubModule_avg_temp : Outport  Port=2
  wires:
  Cell9/2(Cell_temp) -> Add1/9
  [Cell_Current] -> Cell8/1(Cell_Current)
  Cell13/1(Cell_Voltage) -> Add/13
  Cell4/1(Cell_Voltage) -> Add/4
  Module_Current/1 -> [Cell_Current]
  Cell15/1(Cell_Voltage) -> Add/15
  [Cell_Current] -> Cell7/1(Cell_Current)
  [Cell_Current] -> Cell10/1(Cell_Current)
  Cell21/2(Cell_temp) -> Add1/21
  Cell5/1(Cell_Voltage) -> Add/5
  [Cell_Current] -> Cell1/1(Cell_Current)
  Cell2/1(Cell_Voltage) -> Add/2
  Cell19/1(Cell_Voltage) -> Add/19
  [Cell_Current] -> Cell5/1(Cell_Current)
  [Cell_Current] -> Cell11/1(Cell_Current)
  Cell6/1(Cell_Voltage) -> Add/6
  Cell11/1(Cell_Voltage) -> Add/11
  [Cell_Current] -> Cell18/1(Cell_Current)
  Cell7/2(Cell_temp) -> Add1/7
  [Cell_Current] -> Cell21/1(Cell_Current)
  [Cell_Current] -> Cell12/1(Cell_Current)
  [Cell_Current] -> Cell4/1(Cell_Current)
  Cell18/1(Cell_Voltage) -> Add/18
  Cell20/1(Cell_Voltage) -> Add/20
  Cell11/2(Cell_temp) -> Add1/11
  [Cell_Current] -> Cell2/1(Cell_Current)
  Cell16/2(Cell_temp) -> Add1/16
  [Cell_Current] -> Cell15/1(Cell_Current)
  [Cell_Current] -> Cell6/1(Cell_Current)
  [Cell_Current] -> Cell13/1(Cell_Current)
  Cell2/2(Cell_temp) -> Add1/2
  Cell22/2(Cell_temp) -> Add1/22
  Cell9/1(Cell_Voltage) -> Add/9
  Cell7/1(Cell_Voltage) -> Add/7
  [Cell_Current] -> Cell9/1(Cell_Current)
  Cell14/2(Cell_temp) -> Add1/14
  Cell17/1(Cell_Voltage) -> Add/17
  Cell10/2(Cell_temp) -> Add1/10
  [Cell_Current] -> Cell16/1(Cell_Current)
  Cell8/1(Cell_Voltage) -> Add/8
  Cell21/1(Cell_Voltage) -> Add/21
  Cell12/2(Cell_temp) -> Add1/12
  Cell22/1(Cell_Voltage) -> Add/22
  [Cell_Current] -> Cell20/1(Cell_Current)
  [Cell_Current] -> Cell17/1(Cell_Current)
  Cell10/1(Cell_Voltage) -> Add/10
  Cell18/2(Cell_temp) -> Add1/18
  Cell14/1(Cell_Voltage) -> Add/14
  Cell16/1(Cell_Voltage) -> Add/16
  [Cell_Current] -> Cell3/1(Cell_Current)
  Cell12/1(Cell_Voltage) -> Add/12
  Cell20/2(Cell_temp) -> Add1/20
  Cell1/1(Cell_Voltage) -> Add/1
  [Cell_Current] -> Cell19/1(Cell_Current)
  Cell3/1(Cell_Voltage) -> Add/3
  [Cell_Current] -> Cell22/1(Cell_Current)
  [Cell_Current] -> Cell14/1(Cell_Current)
  Cell19/2(Cell_temp) -> Add1/19
  Cell6/2(Cell_temp) -> Add1/6
  Cell17/2(Cell_temp) -> Add1/17
  Cell15/2(Cell_temp) -> Add1/15
  Cell8/2(Cell_temp) -> Add1/8
  Cell3/2(Cell_temp) -> Add1/3
  Cell13/2(Cell_temp) -> Add1/13
  Add/1 -> SubModule_Voltage/1
  Cell4/2(Cell_temp) -> Add1/4
  Cell5/2(Cell_temp) -> Add1/5
  Cell1/2(Cell_temp) -> Add1/1
  Add1/1 -> Divide/1
  Constant/1 -> Divide/2
  Divide/1 -> SubModule_avg_temp/1
  [Cell_Current] -> Cell24/1(Cell_Current)
  [Cell_Current] -> Cell23/1(Cell_Current)
  Cell23/1(Cell_Voltage) -> Add/23
  Cell24/1(Cell_Voltage) -> Add/24
  Cell23/2(Cell_temp) -> Add1/23
  Cell24/2(Cell_temp) -> Add1/24

== system System3/Battery2/SOCEstimator/SOCEstimator ==
  SOC_Initial : Inport
  Current : Inport  Port=2
  CellCapacity : Inport  Port=3
  Add1 : Sum  Inputs=+-
  Constant : Constant  Value=100  SampleTime=-1
  Constant1 : Constant  Value=3600  SampleTime=-1
  Delay : Delay  DelayLength=1  InitialConditionSource=Input port
      settings: InputPortMap=u0,p4
  Divide : Product  Inputs=*//
  Divide1 : Product  Inputs=*/
  Integrator : Integrator
  Saturation1 : Saturate  UpperLimit=1  LowerLimit=0
  SOC : Outport
  wires:
  Add1/1 -> Saturation1/1
  Constant/1 -> Divide1/2
  Divide1/1 -> Delay/2, Add1/1
  Divide/1 -> Add1/2
  Saturation1/1 -> Delay/1
  SOC_Initial/1 -> Divide1/1
  Current/1 -> Integrator/1
  Delay/1 -> SOC/1
  CellCapacity/1 -> Divide/2
  Constant1/1 -> Divide/3
  Integrator/1 -> Divide/1

== system System3/Battery1/Module1/SubModule_1/Cell1 ==
  Cell_Current : Inport
  2RC : Subsystem
  Add : Sum  Inputs=---+
  Lookup Table Dynamic2 : simulink/Lookup Tables/Lookup Table Dynamic  LookUpMeth=Interpolation-Use End Values  OutDataType=fixdt('double')  OutScaling=[]  OutputDataTypeScalingMode=Specify via dialog  OutDataTypeStr=fixdt('double')  DoSatur=off
  Product : Product
  Redution_factor : Constant  Value=[0.8 0.85 0.88 0.95 1 0.98 0.95]
  SOCEstimator : Subsystem  TreatAsAtomicUnit=on
  SOC_Mapping : Subsystem
  Scope : Scope
      settings: DataLoggingSaveFormat=Array
  Scope1 : Scope
      settings: DataLoggingVariableName=ScopeData2  DataLoggingSaveFormat=Array
  Scope2 : Scope
      settings: DataLoggingSaveFormat=Array
  Subsystem : Subsystem
  Temp : Constant  Value=[0 10 20 30 40 50 60]
  Cell_Voltage : Outport
  Cell_temp : Outport  Port=2
  wires:
  2RC/2(V2) -> Add/2
  SOC_Mapping/3(C1) -> 2RC/4(C1)
  SOCEstimator/1(SOC) -> SOC_Mapping/1(SOC), Scope/1
  Add/1 -> Scope2/1, Cell_Voltage/1
  SOC_Mapping/1(Ri) -> Subsystem/2(Ri), 2RC/2(Ri)
  2RC/1(V1) -> Add/1
  2RC/3(Vi) -> Add/3
  Cell_Current/1 -> Subsystem/1(Cell_Current), 2RC/1(Current), SOCEstimator/2(Current)
  SOC_Mapping/2(R1) -> 2RC/3(R1)
  [Cell_Capacity] -> Product/1
  SOC_Mapping/5(C2) -> 2RC/6(C2)
  SOC_Mapping/4(R2) -> 2RC/5(R2)
  [SOC_Iinitial] -> SOCEstimator/1(SOC_Initial)
  SOC_Mapping/6(OCV) -> Add/4
  Subsystem/1(Temp_Cell) -> Scope1/1, SOC_Mapping/2(Cell_Temp), Lookup Table Dynamic2/1, Cell_temp/1
  Product/1 -> SOCEstimator/3(Cell_Capacity)
  Lookup Table Dynamic2/1 -> Product/2
  Temp/1 -> Lookup Table Dynamic2/2
  Redution_factor/1 -> Lookup Table Dynamic2/3

== system System3/Battery1/Module1/SubModule_1/Cell10 ==
  Cell_Current : Inport
  2RC : Subsystem
  Add : Sum  Inputs=---+
  Lookup Table Dynamic2 : simulink/Lookup Tables/Lookup Table Dynamic  LookUpMeth=Interpolation-Use End Values  OutDataType=fixdt('double')  OutScaling=[]  OutputDataTypeScalingMode=Specify via dialog  OutDataTypeStr=fixdt('double')  DoSatur=off
  Product : Product
  Redution_factor : Constant  Value=[0.8 0.85 0.88 0.95 1 0.98 0.95]
  SOCEstimator : Subsystem  TreatAsAtomicUnit=on
  SOC_Mapping : Subsystem
  Scope : Scope
      settings: DataLoggingSaveFormat=Array
  Scope1 : Scope
      settings: DataLoggingVariableName=ScopeData2  DataLoggingSaveFormat=Array
  Scope2 : Scope
      settings: DataLoggingSaveFormat=Array
  Subsystem : Subsystem
  Temp : Constant  Value=[0 10 20 30 40 50 60]
  Cell_Voltage : Outport
  Cell_temp : Outport  Port=2
  wires:
  2RC/2(V2) -> Add/2
  SOC_Mapping/3(C1) -> 2RC/4(C1)
  SOCEstimator/1(SOC) -> SOC_Mapping/1(SOC), Scope/1
  Add/1 -> Scope2/1, Cell_Voltage/1
  SOC_Mapping/1(Ri) -> Subsystem/2(Ri), 2RC/2(Ri)
  2RC/1(V1) -> Add/1
  2RC/3(Vi) -> Add/3
  Cell_Current/1 -> Subsystem/1(Cell_Current), 2RC/1(Current), SOCEstimator/2(Current)
  SOC_Mapping/2(R1) -> 2RC/3(R1)
  [Cell_Capacity] -> Product/1
  SOC_Mapping/5(C2) -> 2RC/6(C2)
  SOC_Mapping/4(R2) -> 2RC/5(R2)
  [SOC_Iinitial] -> SOCEstimator/1(SOC_Initial)
  SOC_Mapping/6(OCV) -> Add/4
  Subsystem/1(Temp_Cell) -> Scope1/1, SOC_Mapping/2(Cell_Temp), Lookup Table Dynamic2/1, Cell_temp/1
  Product/1 -> SOCEstimator/3(Cell_Capacity)
  Lookup Table Dynamic2/1 -> Product/2
  Temp/1 -> Lookup Table Dynamic2/2
  Redution_factor/1 -> Lookup Table Dynamic2/3

== system System3/Battery1/Module1/SubModule_1/Cell11 ==
  Cell_Current : Inport
  2RC : Subsystem
  Add : Sum  Inputs=---+
  Lookup Table Dynamic2 : simulink/Lookup Tables/Lookup Table Dynamic  LookUpMeth=Interpolation-Use End Values  OutDataType=fixdt('double')  OutScaling=[]  OutputDataTypeScalingMode=Specify via dialog  OutDataTypeStr=fixdt('double')  DoSatur=off
  Product : Product
  Redution_factor : Constant  Value=[0.8 0.85 0.88 0.95 1 0.98 0.95]
  SOCEstimator : Subsystem  TreatAsAtomicUnit=on
  SOC_Mapping : Subsystem
  Scope : Scope
      settings: DataLoggingSaveFormat=Array
  Scope1 : Scope
      settings: DataLoggingVariableName=ScopeData2  DataLoggingSaveFormat=Array
  Scope2 : Scope
      settings: DataLoggingSaveFormat=Array
  Subsystem : Subsystem
  Temp : Constant  Value=[0 10 20 30 40 50 60]
  Cell_Voltage : Outport
  Cell_temp : Outport  Port=2
  wires:
  Redution_factor/1 -> Lookup Table Dynamic2/3
  Temp/1 -> Lookup Table Dynamic2/2
  Lookup Table Dynamic2/1 -> Product/2
  Product/1 -> SOCEstimator/3(Cell_Capacity)
  Subsystem/1(Temp_Cell) -> Cell_temp/1, Lookup Table Dynamic2/1, SOC_Mapping/2(Cell_Temp), Scope1/1
  SOC_Mapping/6(OCV) -> Add/4
  [SOC_Iinitial] -> SOCEstimator/1(SOC_Initial)
  SOC_Mapping/4(R2) -> 2RC/5(R2)
  SOC_Mapping/5(C2) -> 2RC/6(C2)
  [Cell_Capacity] -> Product/1
  SOC_Mapping/2(R1) -> 2RC/3(R1)
  Cell_Current/1 -> SOCEstimator/2(Current), 2RC/1(Current), Subsystem/1(Cell_Current)
  2RC/3(Vi) -> Add/3
  2RC/1(V1) -> Add/1
  SOC_Mapping/1(Ri) -> 2RC/2(Ri), Subsystem/2(Ri)
  Add/1 -> Cell_Voltage/1, Scope2/1
  SOCEstimator/1(SOC) -> Scope/1, SOC_Mapping/1(SOC)
  SOC_Mapping/3(C1) -> 2RC/4(C1)
  2RC/2(V2) -> Add/2

== system System3/Battery1/Module1/SubModule_1/Cell12 ==
  Cell_Current : Inport
  2RC : Subsystem
  Add : Sum  Inputs=---+
  Lookup Table Dynamic2 : simulink/Lookup Tables/Lookup Table Dynamic  LookUpMeth=Interpolation-Use End Values  OutDataType=fixdt('double')  OutScaling=[]  OutputDataTypeScalingMode=Specify via dialog  OutDataTypeStr=fixdt('double')  DoSatur=off
  Product : Product
  Redution_factor : Constant  Value=[0.8 0.85 0.88 0.95 1 0.98 0.95]
  SOCEstimator : Subsystem  TreatAsAtomicUnit=on
  SOC_Mapping : Subsystem
  Scope : Scope
      settings: DataLoggingSaveFormat=Array
  Scope1 : Scope
      settings: DataLoggingVariableName=ScopeData2  DataLoggingSaveFormat=Array
  Scope2 : Scope
      settings: DataLoggingSaveFormat=Array
  Subsystem : Subsystem
  Temp : Constant  Value=[0 10 20 30 40 50 60]
  Cell_Voltage : Outport
  Cell_temp : Outport  Port=2
  wires:
  2RC/2(V2) -> Add/2
  SOC_Mapping/3(C1) -> 2RC/4(C1)
  SOCEstimator/1(SOC) -> SOC_Mapping/1(SOC), Scope/1
  Add/1 -> Scope2/1, Cell_Voltage/1
  SOC_Mapping/1(Ri) -> Subsystem/2(Ri), 2RC/2(Ri)
  2RC/1(V1) -> Add/1
  2RC/3(Vi) -> Add/3
  Cell_Current/1 -> Subsystem/1(Cell_Current), 2RC/1(Current), SOCEstimator/2(Current)
  SOC_Mapping/2(R1) -> 2RC/3(R1)
  [Cell_Capacity] -> Product/1
  SOC_Mapping/5(C2) -> 2RC/6(C2)
  SOC_Mapping/4(R2) -> 2RC/5(R2)
  [SOC_Iinitial] -> SOCEstimator/1(SOC_Initial)
  SOC_Mapping/6(OCV) -> Add/4
  Subsystem/1(Temp_Cell) -> Scope1/1, SOC_Mapping/2(Cell_Temp), Lookup Table Dynamic2/1, Cell_temp/1
  Product/1 -> SOCEstimator/3(Cell_Capacity)
  Lookup Table Dynamic2/1 -> Product/2
  Temp/1 -> Lookup Table Dynamic2/2
  Redution_factor/1 -> Lookup Table Dynamic2/3

== system System3/Battery1/Module1/SubModule_1/Cell13 ==
  Cell_Current : Inport
  2RC : Subsystem
  Add : Sum  Inputs=---+
  Lookup Table Dynamic2 : simulink/Lookup Tables/Lookup Table Dynamic  LookUpMeth=Interpolation-Use End Values  OutDataType=fixdt('double')  OutScaling=[]  OutputDataTypeScalingMode=Specify via dialog  OutDataTypeStr=fixdt('double')  DoSatur=off
  Product : Product
  Redution_factor : Constant  Value=[0.8 0.85 0.88 0.95 1 0.98 0.95]
  SOCEstimator : Subsystem  TreatAsAtomicUnit=on
  SOC_Mapping : Subsystem
  Scope : Scope
      settings: DataLoggingSaveFormat=Array
  Scope1 : Scope
      settings: DataLoggingVariableName=ScopeData2  DataLoggingSaveFormat=Array
  Scope2 : Scope
      settings: DataLoggingSaveFormat=Array
  Subsystem : Subsystem
  Temp : Constant  Value=[0 10 20 30 40 50 60]
  Cell_Voltage : Outport
  Cell_temp : Outport  Port=2
  wires:
  Redution_factor/1 -> Lookup Table Dynamic2/3
  Temp/1 -> Lookup Table Dynamic2/2
  Lookup Table Dynamic2/1 -> Product/2
  Product/1 -> SOCEstimator/3(Cell_Capacity)
  Subsystem/1(Temp_Cell) -> Cell_temp/1, Lookup Table Dynamic2/1, SOC_Mapping/2(Cell_Temp), Scope1/1
  SOC_Mapping/6(OCV) -> Add/4
  [SOC_Iinitial] -> SOCEstimator/1(SOC_Initial)
  SOC_Mapping/4(R2) -> 2RC/5(R2)
  SOC_Mapping/5(C2) -> 2RC/6(C2)
  [Cell_Capacity] -> Product/1
  SOC_Mapping/2(R1) -> 2RC/3(R1)
  Cell_Current/1 -> SOCEstimator/2(Current), 2RC/1(Current), Subsystem/1(Cell_Current)
  2RC/3(Vi) -> Add/3
  2RC/1(V1) -> Add/1
  SOC_Mapping/1(Ri) -> 2RC/2(Ri), Subsystem/2(Ri)
  Add/1 -> Cell_Voltage/1, Scope2/1
  SOCEstimator/1(SOC) -> Scope/1, SOC_Mapping/1(SOC)
  SOC_Mapping/3(C1) -> 2RC/4(C1)
  2RC/2(V2) -> Add/2

== system System3/Battery1/Module1/SubModule_1/Cell14 ==
  Cell_Current : Inport
  2RC : Subsystem
  Add : Sum  Inputs=---+
  Lookup Table Dynamic2 : simulink/Lookup Tables/Lookup Table Dynamic  LookUpMeth=Interpolation-Use End Values  OutDataType=fixdt('double')  OutScaling=[]  OutputDataTypeScalingMode=Specify via dialog  OutDataTypeStr=fixdt('double')  DoSatur=off
  Product : Product
  Redution_factor : Constant  Value=[0.8 0.85 0.88 0.95 1 0.98 0.95]
  SOCEstimator : Subsystem  TreatAsAtomicUnit=on
  SOC_Mapping : Subsystem
  Scope : Scope
      settings: DataLoggingSaveFormat=Array
  Scope1 : Scope
      settings: DataLoggingVariableName=ScopeData2  DataLoggingSaveFormat=Array
  Scope2 : Scope
      settings: DataLoggingSaveFormat=Array
  Subsystem : Subsystem
  Temp : Constant  Value=[0 10 20 30 40 50 60]
  Cell_Voltage : Outport
  Cell_temp : Outport  Port=2
  wires:
  Redution_factor/1 -> Lookup Table Dynamic2/3
  Temp/1 -> Lookup Table Dynamic2/2
  Lookup Table Dynamic2/1 -> Product/2
  Product/1 -> SOCEstimator/3(Cell_Capacity)
  Subsystem/1(Temp_Cell) -> Cell_temp/1, Lookup Table Dynamic2/1, SOC_Mapping/2(Cell_Temp), Scope1/1
  SOC_Mapping/6(OCV) -> Add/4
  [SOC_Iinitial] -> SOCEstimator/1(SOC_Initial)
  SOC_Mapping/4(R2) -> 2RC/5(R2)
  SOC_Mapping/5(C2) -> 2RC/6(C2)
  [Cell_Capacity] -> Product/1
  SOC_Mapping/2(R1) -> 2RC/3(R1)
  Cell_Current/1 -> SOCEstimator/2(Current), 2RC/1(Current), Subsystem/1(Cell_Current)
  2RC/3(Vi) -> Add/3
  2RC/1(V1) -> Add/1
  SOC_Mapping/1(Ri) -> 2RC/2(Ri), Subsystem/2(Ri)
  Add/1 -> Cell_Voltage/1, Scope2/1
  SOCEstimator/1(SOC) -> Scope/1, SOC_Mapping/1(SOC)
  SOC_Mapping/3(C1) -> 2RC/4(C1)
  2RC/2(V2) -> Add/2

== system System3/Battery1/Module1/SubModule_1/Cell15 ==
  Cell_Current : Inport
  2RC : Subsystem
  Add : Sum  Inputs=---+
  Lookup Table Dynamic2 : simulink/Lookup Tables/Lookup Table Dynamic  LookUpMeth=Interpolation-Use End Values  OutDataType=fixdt('double')  OutScaling=[]  OutputDataTypeScalingMode=Specify via dialog  OutDataTypeStr=fixdt('double')  DoSatur=off
  Product : Product
  Redution_factor : Constant  Value=[0.8 0.85 0.88 0.95 1 0.98 0.95]
  SOCEstimator : Subsystem  TreatAsAtomicUnit=on
  SOC_Mapping : Subsystem
  Scope : Scope
      settings: DataLoggingSaveFormat=Array
  Scope1 : Scope
      settings: DataLoggingVariableName=ScopeData2  DataLoggingSaveFormat=Array
  Scope2 : Scope
      settings: DataLoggingSaveFormat=Array
  Subsystem : Subsystem
  Temp : Constant  Value=[0 10 20 30 40 50 60]
  Cell_Voltage : Outport
  Cell_temp : Outport  Port=2
  wires:
  Redution_factor/1 -> Lookup Table Dynamic2/3
  Temp/1 -> Lookup Table Dynamic2/2
  Lookup Table Dynamic2/1 -> Product/2
  Product/1 -> SOCEstimator/3(Cell_Capacity)
  Subsystem/1(Temp_Cell) -> Cell_temp/1, Lookup Table Dynamic2/1, SOC_Mapping/2(Cell_Temp), Scope1/1
  SOC_Mapping/6(OCV) -> Add/4
  [SOC_Iinitial] -> SOCEstimator/1(SOC_Initial)
  SOC_Mapping/4(R2) -> 2RC/5(R2)
  SOC_Mapping/5(C2) -> 2RC/6(C2)
  [Cell_Capacity] -> Product/1
  SOC_Mapping/2(R1) -> 2RC/3(R1)
  Cell_Current/1 -> SOCEstimator/2(Current), 2RC/1(Current), Subsystem/1(Cell_Current)
  2RC/3(Vi) -> Add/3
  2RC/1(V1) -> Add/1
  SOC_Mapping/1(Ri) -> 2RC/2(Ri), Subsystem/2(Ri)
  Add/1 -> Cell_Voltage/1, Scope2/1
  SOCEstimator/1(SOC) -> Scope/1, SOC_Mapping/1(SOC)
  SOC_Mapping/3(C1) -> 2RC/4(C1)
  2RC/2(V2) -> Add/2

== system System3/Battery1/Module1/SubModule_1/Cell16 ==
  Cell_Current : Inport
  2RC : Subsystem
  Add : Sum  Inputs=---+
  Lookup Table Dynamic2 : simulink/Lookup Tables/Lookup Table Dynamic  LookUpMeth=Interpolation-Use End Values  OutDataType=fixdt('double')  OutScaling=[]  OutputDataTypeScalingMode=Specify via dialog  OutDataTypeStr=fixdt('double')  DoSatur=off
  Product : Product
  Redution_factor : Constant  Value=[0.8 0.85 0.88 0.95 1 0.98 0.95]
  SOCEstimator : Subsystem  TreatAsAtomicUnit=on
  SOC_Mapping : Subsystem
  Scope : Scope
      settings: DataLoggingSaveFormat=Array
  Scope1 : Scope
      settings: DataLoggingVariableName=ScopeData2  DataLoggingSaveFormat=Array
  Scope2 : Scope
      settings: DataLoggingSaveFormat=Array
  Subsystem : Subsystem
  Temp : Constant  Value=[0 10 20 30 40 50 60]
  Cell_Voltage : Outport
  Cell_temp : Outport  Port=2
  wires:
  Redution_factor/1 -> Lookup Table Dynamic2/3
  Temp/1 -> Lookup Table Dynamic2/2
  Lookup Table Dynamic2/1 -> Product/2
  Product/1 -> SOCEstimator/3(Cell_Capacity)
  Subsystem/1(Temp_Cell) -> Cell_temp/1, Lookup Table Dynamic2/1, SOC_Mapping/2(Cell_Temp), Scope1/1
  SOC_Mapping/6(OCV) -> Add/4
  [SOC_Iinitial] -> SOCEstimator/1(SOC_Initial)
  SOC_Mapping/4(R2) -> 2RC/5(R2)
  SOC_Mapping/5(C2) -> 2RC/6(C2)
  [Cell_Capacity] -> Product/1
  SOC_Mapping/2(R1) -> 2RC/3(R1)
  Cell_Current/1 -> SOCEstimator/2(Current), 2RC/1(Current), Subsystem/1(Cell_Current)
  2RC/3(Vi) -> Add/3
  2RC/1(V1) -> Add/1
  SOC_Mapping/1(Ri) -> 2RC/2(Ri), Subsystem/2(Ri)
  Add/1 -> Cell_Voltage/1, Scope2/1
  SOCEstimator/1(SOC) -> Scope/1, SOC_Mapping/1(SOC)
  SOC_Mapping/3(C1) -> 2RC/4(C1)
  2RC/2(V2) -> Add/2

== system System3/Battery1/Module1/SubModule_1/Cell17 ==
  Cell_Current : Inport
  2RC : Subsystem
  Add : Sum  Inputs=---+
  Lookup Table Dynamic2 : simulink/Lookup Tables/Lookup Table Dynamic  LookUpMeth=Interpolation-Use End Values  OutDataType=fixdt('double')  OutScaling=[]  OutputDataTypeScalingMode=Specify via dialog  OutDataTypeStr=fixdt('double')  DoSatur=off
  Product : Product
  Redution_factor : Constant  Value=[0.8 0.85 0.88 0.95 1 0.98 0.95]
  SOCEstimator : Subsystem  TreatAsAtomicUnit=on
  SOC_Mapping : Subsystem
  Scope : Scope
      settings: DataLoggingSaveFormat=Array
  Scope1 : Scope
      settings: DataLoggingVariableName=ScopeData2  DataLoggingSaveFormat=Array
  Scope2 : Scope
      settings: DataLoggingSaveFormat=Array
  Subsystem : Subsystem
  Temp : Constant  Value=[0 10 20 30 40 50 60]
  Cell_Voltage : Outport
  Cell_temp : Outport  Port=2
  wires:
  2RC/2(V2) -> Add/2
  SOC_Mapping/3(C1) -> 2RC/4(C1)
  SOCEstimator/1(SOC) -> SOC_Mapping/1(SOC), Scope/1
  Add/1 -> Scope2/1, Cell_Voltage/1
  SOC_Mapping/1(Ri) -> Subsystem/2(Ri), 2RC/2(Ri)
  2RC/1(V1) -> Add/1
  2RC/3(Vi) -> Add/3
  Cell_Current/1 -> Subsystem/1(Cell_Current), 2RC/1(Current), SOCEstimator/2(Current)
  SOC_Mapping/2(R1) -> 2RC/3(R1)
  [Cell_Capacity] -> Product/1
  SOC_Mapping/5(C2) -> 2RC/6(C2)
  SOC_Mapping/4(R2) -> 2RC/5(R2)
  [SOC_Iinitial] -> SOCEstimator/1(SOC_Initial)
  SOC_Mapping/6(OCV) -> Add/4
  Subsystem/1(Temp_Cell) -> Scope1/1, SOC_Mapping/2(Cell_Temp), Lookup Table Dynamic2/1, Cell_temp/1
  Product/1 -> SOCEstimator/3(Cell_Capacity)
  Lookup Table Dynamic2/1 -> Product/2
  Temp/1 -> Lookup Table Dynamic2/2
  Redution_factor/1 -> Lookup Table Dynamic2/3

== system System3/Battery1/Module1/SubModule_1/Cell18 ==
  Cell_Current : Inport
  2RC : Subsystem
  Add : Sum  Inputs=---+
  Lookup Table Dynamic2 : simulink/Lookup Tables/Lookup Table Dynamic  LookUpMeth=Interpolation-Use End Values  OutDataType=fixdt('double')  OutScaling=[]  OutputDataTypeScalingMode=Specify via dialog  OutDataTypeStr=fixdt('double')  DoSatur=off
  Product : Product
  Redution_factor : Constant  Value=[0.8 0.85 0.88 0.95 1 0.98 0.95]
  SOCEstimator : Subsystem  TreatAsAtomicUnit=on
  SOC_Mapping : Subsystem
  Scope : Scope
      settings: DataLoggingSaveFormat=Array
  Scope1 : Scope
      settings: DataLoggingVariableName=ScopeData2  DataLoggingSaveFormat=Array
  Scope2 : Scope
      settings: DataLoggingSaveFormat=Array
  Subsystem : Subsystem
  Temp : Constant  Value=[0 10 20 30 40 50 60]
  Cell_Voltage : Outport
  Cell_temp : Outport  Port=2
  wires:
  Redution_factor/1 -> Lookup Table Dynamic2/3
  Temp/1 -> Lookup Table Dynamic2/2
  Lookup Table Dynamic2/1 -> Product/2
  Product/1 -> SOCEstimator/3(Cell_Capacity)
  Subsystem/1(Temp_Cell) -> Cell_temp/1, Lookup Table Dynamic2/1, SOC_Mapping/2(Cell_Temp), Scope1/1
  SOC_Mapping/6(OCV) -> Add/4
  [SOC_Iinitial] -> SOCEstimator/1(SOC_Initial)
  SOC_Mapping/4(R2) -> 2RC/5(R2)
  SOC_Mapping/5(C2) -> 2RC/6(C2)
  [Cell_Capacity] -> Product/1
  SOC_Mapping/2(R1) -> 2RC/3(R1)
  Cell_Current/1 -> SOCEstimator/2(Current), 2RC/1(Current), Subsystem/1(Cell_Current)
  2RC/3(Vi) -> Add/3
  2RC/1(V1) -> Add/1
  SOC_Mapping/1(Ri) -> 2RC/2(Ri), Subsystem/2(Ri)
  Add/1 -> Cell_Voltage/1, Scope2/1
  SOCEstimator/1(SOC) -> Scope/1, SOC_Mapping/1(SOC)
  SOC_Mapping/3(C1) -> 2RC/4(C1)
  2RC/2(V2) -> Add/2

== system System3/Battery1/Module1/SubModule_1/Cell19 ==
  Cell_Current : Inport
  2RC : Subsystem
  Add : Sum  Inputs=---+
  Lookup Table Dynamic2 : simulink/Lookup Tables/Lookup Table Dynamic  LookUpMeth=Interpolation-Use End Values  OutDataType=fixdt('double')  OutScaling=[]  OutputDataTypeScalingMode=Specify via dialog  OutDataTypeStr=fixdt('double')  DoSatur=off
  Product : Product
  Redution_factor : Constant  Value=[0.8 0.85 0.88 0.95 1 0.98 0.95]
  SOCEstimator : Subsystem  TreatAsAtomicUnit=on
  SOC_Mapping : Subsystem
  Scope : Scope
      settings: DataLoggingSaveFormat=Array
  Scope1 : Scope
      settings: DataLoggingVariableName=ScopeData2  DataLoggingSaveFormat=Array
  Scope2 : Scope
      settings: DataLoggingSaveFormat=Array
  Subsystem : Subsystem
  Temp : Constant  Value=[0 10 20 30 40 50 60]
  Cell_Voltage : Outport
  Cell_temp : Outport  Port=2
  wires:
  2RC/2(V2) -> Add/2
  SOC_Mapping/3(C1) -> 2RC/4(C1)
  SOCEstimator/1(SOC) -> SOC_Mapping/1(SOC), Scope/1
  Add/1 -> Scope2/1, Cell_Voltage/1
  SOC_Mapping/1(Ri) -> Subsystem/2(Ri), 2RC/2(Ri)
  2RC/1(V1) -> Add/1
  2RC/3(Vi) -> Add/3
  Cell_Current/1 -> Subsystem/1(Cell_Current), 2RC/1(Current), SOCEstimator/2(Current)
  SOC_Mapping/2(R1) -> 2RC/3(R1)
  [Cell_Capacity] -> Product/1
  SOC_Mapping/5(C2) -> 2RC/6(C2)
  SOC_Mapping/4(R2) -> 2RC/5(R2)
  [SOC_Iinitial] -> SOCEstimator/1(SOC_Initial)
  SOC_Mapping/6(OCV) -> Add/4
  Subsystem/1(Temp_Cell) -> Scope1/1, SOC_Mapping/2(Cell_Temp), Lookup Table Dynamic2/1, Cell_temp/1
  Product/1 -> SOCEstimator/3(Cell_Capacity)
  Lookup Table Dynamic2/1 -> Product/2
  Temp/1 -> Lookup Table Dynamic2/2
  Redution_factor/1 -> Lookup Table Dynamic2/3

== system System3/Battery1/Module1/SubModule_1/Cell2 ==
  Cell_Current : Inport
  2RC : Subsystem
  Add : Sum  Inputs=---+
  Lookup Table Dynamic2 : simulink/Lookup Tables/Lookup Table Dynamic  LookUpMeth=Interpolation-Use End Values  OutDataType=fixdt('double')  OutScaling=[]  OutputDataTypeScalingMode=Specify via dialog  OutDataTypeStr=fixdt('double')  DoSatur=off
  Product : Product
  Redution_factor : Constant  Value=[0.8 0.85 0.88 0.95 1 0.98 0.95]
  SOCEstimator : Subsystem  TreatAsAtomicUnit=on
  SOC_Mapping : Subsystem
  Scope : Scope
      settings: DataLoggingSaveFormat=Array
  Scope1 : Scope
      settings: DataLoggingVariableName=ScopeData2  DataLoggingSaveFormat=Array
  Scope2 : Scope
      settings: DataLoggingSaveFormat=Array
  Subsystem : Subsystem
  Temp : Constant  Value=[0 10 20 30 40 50 60]
  Cell_Voltage : Outport
  Cell_temp : Outport  Port=2
  wires:
  Redution_factor/1 -> Lookup Table Dynamic2/3
  Temp/1 -> Lookup Table Dynamic2/2
  Lookup Table Dynamic2/1 -> Product/2
  Product/1 -> SOCEstimator/3(Cell_Capacity)
  Subsystem/1(Temp_Cell) -> Cell_temp/1, Lookup Table Dynamic2/1, SOC_Mapping/2(Cell_Temp), Scope1/1
  SOC_Mapping/6(OCV) -> Add/4
  [SOC_Iinitial] -> SOCEstimator/1(SOC_Initial)
  SOC_Mapping/4(R2) -> 2RC/5(R2)
  SOC_Mapping/5(C2) -> 2RC/6(C2)
  [Cell_Capacity] -> Product/1
  SOC_Mapping/2(R1) -> 2RC/3(R1)
  Cell_Current/1 -> SOCEstimator/2(Current), 2RC/1(Current), Subsystem/1(Cell_Current)
  2RC/3(Vi) -> Add/3
  2RC/1(V1) -> Add/1
  SOC_Mapping/1(Ri) -> 2RC/2(Ri), Subsystem/2(Ri)
  Add/1 -> Cell_Voltage/1, Scope2/1
  SOCEstimator/1(SOC) -> Scope/1, SOC_Mapping/1(SOC)
  SOC_Mapping/3(C1) -> 2RC/4(C1)
  2RC/2(V2) -> Add/2
